simulink library "libreria_medidores1T"  (R2018a)
settings: Solver=VariableStepAuto  StartTime=0.0  StopTime=10.0  RelTol=1e-3
undefined symbols (not defined in the file or in its folder): Ts
libraries: powerlib_meascontrol x1
settings Model: Creator=Unalman  LastModifiedBy=ana-n

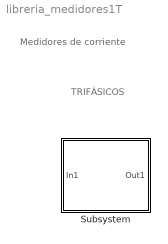
== system libreria_medidores1T ==
  note: TRIFÁSICOS
  note: Medidores de corriente
  Subsystem : Subsystem
      mask Display:
      | port_label('input',1,'Iabc');
      | port_label('output',1,'RMS_3F');

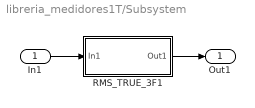
== system libreria_medidores1T/Subsystem ==
  In1 : Inport
  RMS_TRUE_3F1 : Subsystem
      mask Display: color('blue');disp('RMS_TRUE_3F')
  Out1 : Outport
  wires:
  RMS_TRUE_3F1/1(Out1) -> Out1/1
  In1/1 -> RMS_TRUE_3F1/1(In1)

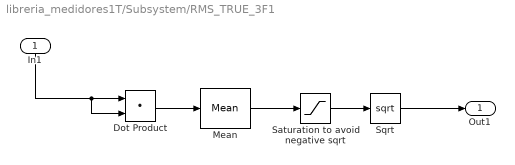
== system libreria_medidores1T/Subsystem/RMS_TRUE_3F1 ==
  In1 : Inport
  Dot Product : DotProduct  InputSameDT=on  OutDataTypeStr=Inherit: Inherit via internal rule
  Mean : powerlib_meascontrol/Measurements/Mean  Freq=60  Vinit=0  Ts=Ts
  Saturation to avoid negative sqrt : Saturate  UpperLimit=Inf  LowerLimit=0
  Sqrt : Sqrt  SaturateOnIntegerOverflow=on
  Out1 : Outport
  wires:
  Sqrt/1 -> Out1/1
  In1/1 -> Dot Product/2, Dot Product/1
  Dot Product/1 -> Mean/1
  Saturation to avoid negative sqrt/1 -> Sqrt/1
  Mean/1 -> Saturation to avoid negative sqrt/1
